simulink subsystem "Shrimple_6dof"  (R2023b)
settings: Solver=VariableStepAuto  StartTime=0.0  StopTime=10.0  RelTol=1e-3
undefined symbols (not defined in the file): Apogee_stop, BG0, Burnout_stop, COM_table, day_seconds, F, HG0, I, include_turbulence, latlong0, launch_elevation, Light, m_table, MIL, MOI_table, time0, turbulence_noise_seeds, uvw0_B, v0_NED, w0_BN, wind_model_type, x0_NED
libraries: sharedtransform x4, simulink_extras x2, aerolibwind2 x1
settings Model: Creator=thatf  LastModifiedBy=thatf

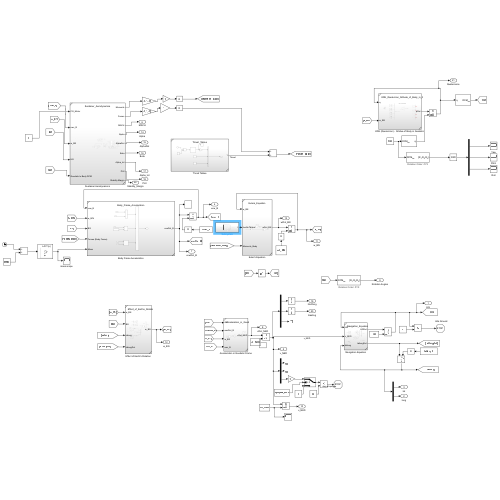
[thumbnail: Simulink's stored preview of the top-level diagram]
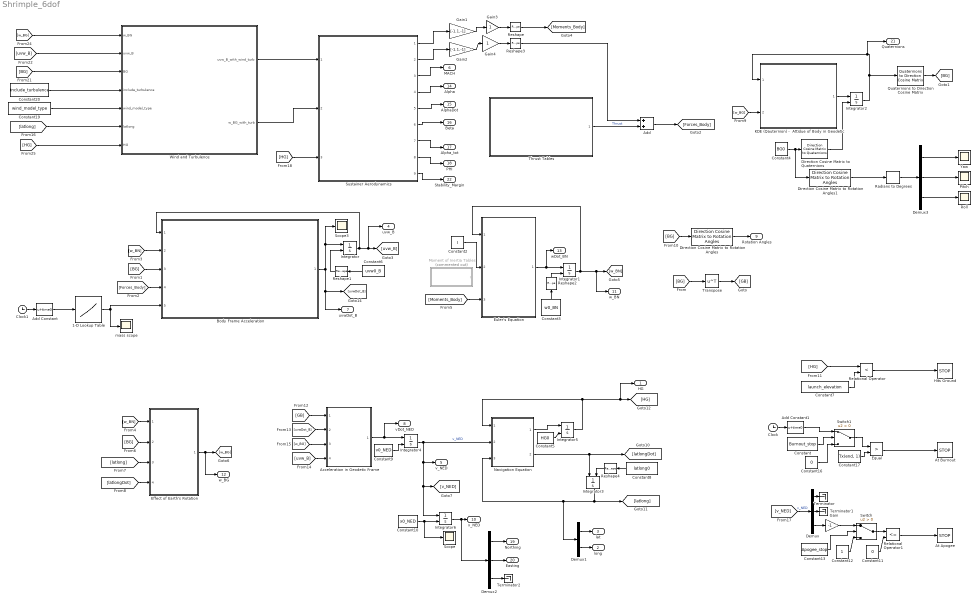
== system Shrimple_6dof ==
  1-D Lookup Table : Lookup_n-D  NumberOfTableDimensions=1  BreakpointsForDimension1=m_table(:,1)  Table=m_table(:,2)  InternalRulePriority=Speed  RndMeth=Simplest
  Acceleration in Geodetic Frame : Subsystem  ReferencedSubsystem=Acceleration_in_Geodetic_Frame
  Add : Sum
  Add Constant : Bias  Bias=time0  SaturateOnIntegerOverflow=off
  Add Constant1 : Bias  Bias=time0  SaturateOnIntegerOverflow=off
  At Apogee : Stop
  At Burnout : Stop
  Body Frame Acceleration : Subsystem  ReferencedSubsystem=Body_Frame_Acceleration
  Clock : Clock
  Clock1 : Clock
  Constant : Constant  Value=Burnout_stop
  Constant10 : Constant  Value=x0_NED
  Constant11 : Constant  Value=0
  Constant12 : Constant
  Constant13 : Constant  Value=Apogee_stop
  Constant16 : Constant  Value=0
  Constant17 : Constant  Value=Tx(end, 1)
  Constant19 : Constant  Value=wind_model_type
  Constant2 : Constant  Value=I
  Constant20 : Constant  Value=include_turbulence
  Constant3 : Constant  Value=w0_BN
  Constant4 : Constant  Value=BG0
  Constant5 : Constant  Value=HG0
  Constant6 : Constant  Value=uvw0_B
  Constant7 : Constant  Value=launch_elevation
  Constant8 : Constant  Value=latlong0
  Constant9 : Constant  Value=v0_NED
  Demux : Demux  Outputs=3
  Demux1 : Demux  Outputs=2
  Demux2 : Demux  Outputs=3
  Demux3 : Demux  Outputs=3
  Direction Cosine Matrix to Rotation Angles : sharedtransform/Direction Cosine Matrix to Rotation Angles  rotationOrder=ZYX  aMode=aMode  action=None  tolerance=eps(2)
  Direction Cosine Matrix to Rotation Angles1 : sharedtransform/Direction Cosine Matrix to Rotation Angles  rotationOrder=ZYX  aMode=aMode  action=None  tolerance=eps(2)
  Direction Cosine Matrix to Quaternions : sharedtransform/Direction Cosine Matrix  to Quaternions  aMode=0  action=None  tolerance=eps(2)
  Effect of Earth's Rotation : Subsystem  ReferencedSubsystem=Effect_of_Earths_Rotation
  Equal : RelationalOperator  Operator=>  OutDataTypeStr=boolean  RndMeth=Simplest  InputSameDT=off
  Euler's Equation : Subsystem  ReferencedSubsystem=Eulers_Equation
  Gain : Gain  Gain=-1
  Gain1 : Gain  Gain=[-1,1,-1]
  Gain2 : Gain  Gain=[-1,1,-1]
  Gain3 : Gain
  Gain4 : Gain
  Hits Ground : Stop
  Integrator{,1..6} (7 alike) : Integrator  InitialConditionSource=external
  "KDE (Qauternion) -  Attidue of Body in Geodetic " : Subsystem  ReferencedSubsystem=KDE_Qauternion_Attitude_of_Body_in_Geodetic
  Moment of Inertia Tables : Subsystem  Commented=on
  Navigation Equation : Subsystem  ReferencedSubsystem=Navigation_Equation
  Pitch : Scope
  Quaternions to Direction Cosine Matrix : sharedtransform/Quaternions to  Direction Cosine Matrix  aMode=aMode
  Radians to Degrees : simulink_extras/Transformations/Radians to Degrees
  Relational Operator : RelationalOperator  Operator=<  OutDataTypeStr=boolean  RndMeth=Simplest  InputSameDT=off
  Relational Operator1 : RelationalOperator  Operator=<=  OutDataTypeStr=boolean  RndMeth=Simplest  InputSameDT=off
  Reshape{,1..3} (4 alike) : Reshape  OutputDimensionality=Customize  OutputDimensions=[3,1]
  Reshape4 : Reshape  OutputDimensionality=Customize  OutputDimensions=[2,1]
  Roll : Scope
  Scope : Scope
  Scope3 : Scope
  Sustainer Aerodynamics : Subsystem  ReferencedSubsystem=Sustainer_Aerodynamics
  Switch : Switch  Criteria=u2 > Threshold  SaturateOnIntegerOverflow=off  InputSameDT=off
  Switch1 : Switch  Criteria=u2 > Threshold  SaturateOnIntegerOverflow=off  InputSameDT=off
  Terminator : Terminator
  Terminator1 : Terminator
  Terminator2 : Terminator
  Thrust Tables : Subsystem  ReferencedSubsystem=Thrust_Tables
  Transpose : Math  Operator=transpose
  Wind and Turbulence : Subsystem
  Yaw : Scope
  mass scope : Scope
  HG : Outport
  long : Outport  Port=2
  lat : Outport  Port=3
  uvw_B : Outport  Port=4
  v_NED : Outport  Port=5
  MACH : Outport  Port=6
  uvwDot_B : Outport  Port=7
  vDot_NED : Outport  Port=8
  Rotation Angles : Outport  Port=9
  x_NED : Outport  Port=10
  w_BN : Outport  Port=11
  w_BG : Outport  Port=12
  wDot_BN : Outport  Port=13
  Alpha : Outport  Port=14
  AlphaDot : Outport  Port=15
  Beta : Outport  Port=16
  Alpha_tot : Outport  Port=17
  PHI : Outport  Port=18
  Northing : Outport  Port=19
  Easting : Outport  Port=20
  Quaternions : Outport  Port=21
  Stability_Margin : Outport  Port=22
  wires:
  Euler's Equation/1 -> Integrator1/1, wDot_BN/1
  Direction Cosine Matrix to Rotation Angles/1 -> Rotation Angles/1
  [BG] -> Direction Cosine Matrix to Rotation Angles/1
  Direction Cosine Matrix to Quaternions/1 -> Integrator2/2
  Constant5/1 -> Integrator5/2
  [BG] -> Transpose/1
  [BG] -> Body Frame Acceleration/3
  [w_BG] -> Acceleration in Geodetic Frame/3
  Reshape/1 -> [Moments_Body]
  Constant6/1 -> Reshape1/1
  Navigation Equation/2 -> Integrator3/1, [latlongDot]
  Integrator2/1 -> Quaternions to Direction Cosine Matrix/1, "KDE (Qauternion) -  Attidue of Body in Geodetic "/1, Quaternions/1
  Constant3/1 -> Reshape2/1
  [BG] -> Effect of Earth's Rotation/2
  [uvw_B] -> Acceleration in Geodetic Frame/4
  [w_BG] -> "KDE (Qauternion) -  Attidue of Body in Geodetic "/2
  Reshape2/1 -> Integrator1/2
  Reshape1/1 -> Integrator/2
  Integrator3/1 -> Navigation Equation/3, Demux1/1, [latlong]
  Acceleration in Geodetic Frame/1 -> Integrator4/1, vDot_NED/1
  Body Frame Acceleration/1 -> Integrator/1, Scope3/1, [uvwDot_B], uvwDot_B/1
  Gain1/1 -> Gain3/1
  Navigation Equation/1 -> Integrator5/1
  Constant4/1 -> Direction Cosine Matrix to Quaternions/1, Direction Cosine Matrix to Rotation Angles1/1
  Integrator5/1 -> Navigation Equation/1, [HG], HG/1
  Gain2/1 -> Gain4/1
  "KDE (Qauternion) -  Attidue of Body in Geodetic "/1 -> Integrator2/1
  [Moments_Body] -> Euler's Equation/3
  [w_BN] -> Effect of Earth's Rotation/1
  Integrator4/1 -> v_NED/1, [v_NED], Integrator6/1, Navigation Equation/2  "v_NED"
  [w_BN] -> Body Frame Acceleration/2
  Integrator/1 -> Body Frame Acceleration/1, [uvw_B], uvw_B/1
  Quaternions to Direction Cosine Matrix/1 -> [BG]
  [uvwDot_B] -> Acceleration in Geodetic Frame/2
  Effect of Earth's Rotation/1 -> [w_BG], w_BG/1
  [GB] -> Acceleration in Geodetic Frame/1
  Transpose/1 -> [GB]
  Relational Operator/1 -> Hits Ground/1
  [Forces_Body] -> Body Frame Acceleration/4
  [latlongDot] -> Effect of Earth's Rotation/4
  Constant7/1 -> Relational Operator/2
  [latlong] -> Effect of Earth's Rotation/3
  Constant9/1 -> Integrator4/2
  Reshape4/1 -> Integrator3/2
  Integrator1/1 -> Euler's Equation/1, [w_BN], w_BN/1
  Constant8/1 -> Reshape4/1
  Demux1/2 -> long/1
  Demux1/1 -> lat/1
  Constant10/1 -> Integrator6/2, Scope/1
  Integrator6/1 -> x_NED/1, Demux2/1
  Reshape3/1 -> Add/1
  Thrust Tables/1 -> Add/2  "Thrust"
  Add/1 -> [Forces_Body]
  1-D Lookup Table/1 -> Body Frame Acceleration/5, mass scope/1
  Gain3/1 -> Reshape/1
  Gain4/1 -> Reshape3/1
  Demux2/3 -> Terminator2/1
  Direction Cosine Matrix to Rotation Angles1/1 -> Radians to Degrees/1
  Demux3/3 -> Roll/1
  Demux3/2 -> Pitch/1
  Radians to Degrees/1 -> Demux3/1
  Demux3/1 -> Yaw/1
  Sustainer Aerodynamics/8 -> PHI/1
  Sustainer Aerodynamics/7 -> Alpha_tot/1
  Sustainer Aerodynamics/6 -> Beta/1
  Sustainer Aerodynamics/5 -> AlphaDot/1
  Sustainer Aerodynamics/4 -> Alpha/1
  Sustainer Aerodynamics/3 -> MACH/1
  Sustainer Aerodynamics/2 -> Gain2/1
  Sustainer Aerodynamics/1 -> Gain1/1
  [HG] -> Sustainer Aerodynamics/3
  Sustainer Aerodynamics/9 -> Stability_Margin/1
  Equal/1 -> At Burnout/1
  Constant/1 -> Switch1/2
  Constant16/1 -> Switch1/3
  Constant17/1 -> Equal/2
  Switch1/1 -> Equal/1
  Add Constant1/1 -> Switch1/1
  Constant2/1 -> Euler's Equation/2
  Demux2/1 -> Northing/1
  Demux2/2 -> Easting/1
  [w_BG] -> Wind and Turbulence/1(w_BG)
  [uvw_B] -> Wind and Turbulence/2(uvw_B)
  [BG] -> Wind and Turbulence/3(BG)
  Constant20/1 -> Wind and Turbulence/4(include_turbulence)
  Constant19/1 -> Wind and Turbulence/5(wind_model_type)
  [latlong] -> Wind and Turbulence/6(latlong)
  [HG] -> Wind and Turbulence/7(HG)
  Wind and Turbulence/1(uvw_B_with_wind_turb) -> Sustainer Aerodynamics/1
  Wind and Turbulence/2(w_BG_with_turb) -> Sustainer Aerodynamics/2
  Clock1/1 -> Add Constant/1
  Add Constant/1 -> 1-D Lookup Table/1
  Clock/1 -> Add Constant1/1
  [HG] -> Relational Operator/1
  [v_NED] -> Demux/1  "v_NED"
  Demux/1 -> Terminator/1
  Constant13/1 -> Switch/2
  Gain/1 -> Switch/1
  Demux/3 -> Gain/1
  Constant12/1 -> Switch/3
  Switch/1 -> Relational Operator1/1
  Demux/2 -> Terminator1/1
  Constant11/1 -> Relational Operator1/2
  Relational Operator1/1 -> At Apogee/1

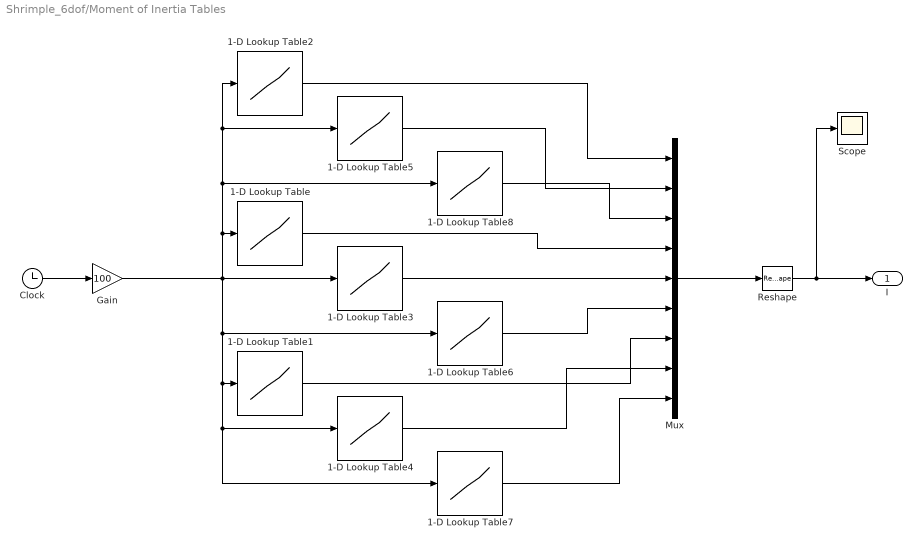
== system Shrimple_6dof/Moment of Inertia Tables ==
  1-D Lookup Table : Lookup_n-D  NumberOfTableDimensions=1  BreakpointsForDimension1=COM_table(:,1)  Table=MOI_table(:,2,1)  InternalRulePriority=Speed  RndMeth=Simplest
  1-D Lookup Table1 : Lookup_n-D  NumberOfTableDimensions=1  BreakpointsForDimension1=COM_table(:,1)  Table=MOI_table(:,3,1)  InternalRulePriority=Speed  RndMeth=Simplest
  1-D Lookup Table2 : Lookup_n-D  NumberOfTableDimensions=1  BreakpointsForDimension1=COM_table(:,1)  Table=MOI_table(:,1,1)  InternalRulePriority=Speed  RndMeth=Simplest
  1-D Lookup Table3 : Lookup_n-D  NumberOfTableDimensions=1  BreakpointsForDimension1=COM_table(:,1)  Table=MOI_table(:,2,2)  InternalRulePriority=Speed  RndMeth=Simplest
  1-D Lookup Table4 : Lookup_n-D  NumberOfTableDimensions=1  BreakpointsForDimension1=COM_table(:,1)  Table=MOI_table(:,3,2)  InternalRulePriority=Speed  RndMeth=Simplest
  1-D Lookup Table5 : Lookup_n-D  NumberOfTableDimensions=1  BreakpointsForDimension1=COM_table(:,1)  Table=MOI_table(:,1,2)  InternalRulePriority=Speed  RndMeth=Simplest
  1-D Lookup Table6 : Lookup_n-D  NumberOfTableDimensions=1  BreakpointsForDimension1=COM_table(:,1)  Table=MOI_table(:,2,3)  InternalRulePriority=Speed  RndMeth=Simplest
  1-D Lookup Table7 : Lookup_n-D  NumberOfTableDimensions=1  BreakpointsForDimension1=COM_table(:,1)  Table=MOI_table(:,3,3)  InternalRulePriority=Speed  RndMeth=Simplest
  1-D Lookup Table8 : Lookup_n-D  NumberOfTableDimensions=1  BreakpointsForDimension1=COM_table(:,1)  Table=MOI_table(:,1,3)  InternalRulePriority=Speed  RndMeth=Simplest
  Clock : Clock
  Gain : Gain  Gain=100
  Mux : Mux  Inputs=9
  Reshape : Reshape  OutputDimensionality=Customize  OutputDimensions=[3,3]
  Scope : Scope
  I : Outport
  wires:
  Gain/1 -> 1-D Lookup Table6/1, 1-D Lookup Table1/1, 1-D Lookup Table4/1, 1-D Lookup Table7/1, 1-D Lookup Table3/1, 1-D Lookup Table/1, 1-D Lookup Table8/1, 1-D Lookup Table5/1, 1-D Lookup Table2/1
  Reshape/1 -> I/1, Scope/1
  Mux/1 -> Reshape/1
  1-D Lookup Table7/1 -> Mux/9
  1-D Lookup Table4/1 -> Mux/8
  1-D Lookup Table1/1 -> Mux/7
  1-D Lookup Table6/1 -> Mux/6
  1-D Lookup Table3/1 -> Mux/5
  1-D Lookup Table/1 -> Mux/4
  1-D Lookup Table8/1 -> Mux/3
  1-D Lookup Table5/1 -> Mux/2
  1-D Lookup Table2/1 -> Mux/1
  Clock/1 -> Gain/1

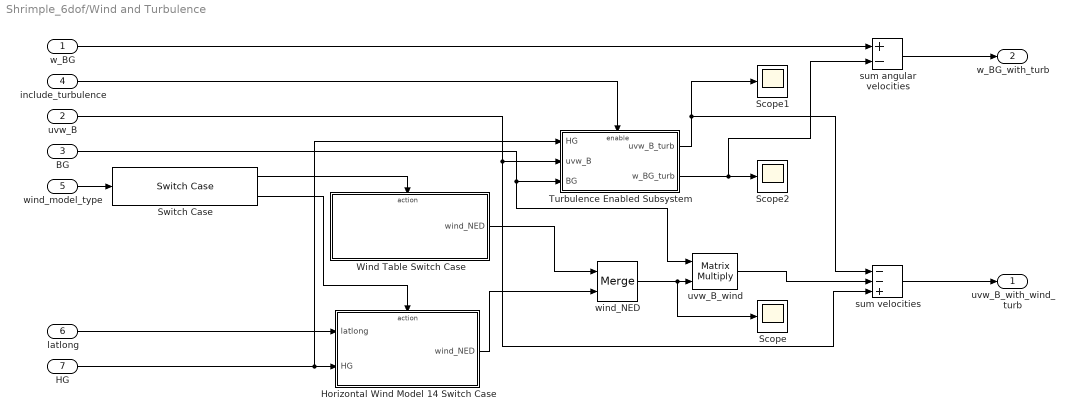
== system Shrimple_6dof/Wind and Turbulence ==
  w_BG : Inport
  uvw_B : Inport  Port=2
  BG : Inport  Port=3
  include_turbulence : Inport  Port=4
  wind_model_type : Inport  Port=5
  latlong : Inport  Port=6
  HG : Inport  Port=7
  Horizontal Wind Model 14 Switch Case : Subsystem  TreatAsAtomicUnit=on
  Scope : Scope
  Scope1 : Scope
  Scope2 : Scope
  Switch Case : SwitchCase  CaseConditions={WindModelType.WindTable, WindModelType.HorizontalWindModel14}  ShowDefaultCase=off
  Turbulence Enabled Subsystem : Subsystem  TreatAsAtomicUnit=on
  Wind Table Switch Case : Subsystem  TreatAsAtomicUnit=on
  sum angular velocities : Sum  Inputs=+-
  sum velocities : Sum  Inputs=--+
  uvw_B_wind : Product  Multiplication=Matrix(*)
  wind_NED : Merge
  uvw_B_with_wind_turb : Outport
  w_BG_with_turb : Outport  Port=2
  wires:
  Turbulence Enabled Subsystem/1(uvw_B_turb) -> sum velocities/1, Scope1/1
  Turbulence Enabled Subsystem/2(w_BG_turb) -> Scope2/1, sum angular velocities/2
  include_turbulence/1 -> Turbulence Enabled Subsystem/Enable
  sum velocities/1 -> uvw_B_with_wind_turb/1
  wind_model_type/1 -> Switch Case/1
  Switch Case/1 -> Wind Table Switch Case/Action
  uvw_B_wind/1 -> sum velocities/2
  Wind Table Switch Case/1(wind_NED) -> wind_NED/1
  w_BG/1 -> sum angular velocities/1
  Horizontal Wind Model 14 Switch Case/1(wind_NED) -> wind_NED/2
  latlong/1 -> Horizontal Wind Model 14 Switch Case/1(latlong)
  wind_NED/1 -> uvw_B_wind/2, Scope/1
  uvw_B/1 -> Turbulence Enabled Subsystem/2(uvw_B), sum velocities/3
  HG/1 -> Horizontal Wind Model 14 Switch Case/2(HG), Turbulence Enabled Subsystem/1(HG)
  Switch Case/2 -> Horizontal Wind Model 14 Switch Case/Action
  sum angular velocities/1 -> w_BG_with_turb/1
  BG/1 -> Turbulence Enabled Subsystem/3(BG), uvw_B_wind/1

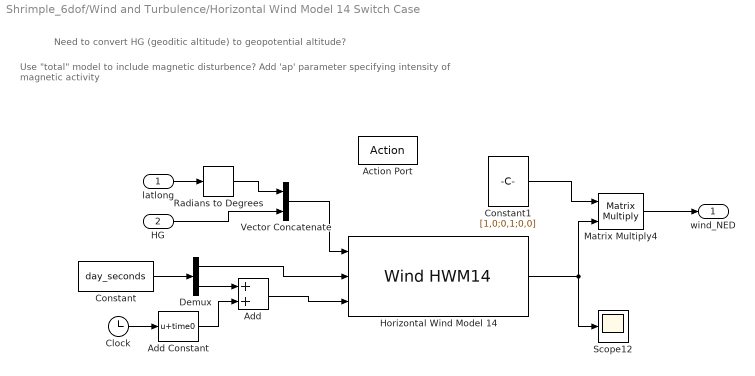
== system Shrimple_6dof/Wind and Turbulence/Horizontal Wind Model 14 Switch Case ==
  note: Need to convert HG (geoditic altitude) to geopotential altitude?
  note: Use "total" model to include magnetic disturbence? Add 'ap' parameter specifying intensity of magnetic activity
  latlong : Inport
  HG : Inport  Port=2
  Action Port : ActionPort
  Add : Sum
  Add Constant : Bias  Bias=time0  SaturateOnIntegerOverflow=off
  Clock : Clock
  Constant : Constant  Value=day_seconds
  Constant1 : Constant  Value=[1,0;0,1;0,0]
  Demux : Demux  Outputs=2
  Horizontal Wind Model 14 : WindHWM14
  Matrix Multiply4 : Product  Multiplication=Matrix(*)
  Radians to Degrees : simulink_extras/Transformations/Radians to Degrees
  Scope12 : Scope
  Vector Concatenate : Concatenate
  wind_NED : Outport
  wires:
  Add Constant/1 -> Add/2
  Clock/1 -> Add Constant/1
  Demux/2 -> Add/1
  Demux/1 -> Horizontal Wind Model 14/2
  Constant/1 -> Demux/1
  Matrix Multiply4/1 -> wind_NED/1
  Constant1/1 -> Matrix Multiply4/1
  Horizontal Wind Model 14/1 -> Scope12/1, Matrix Multiply4/2
  Vector Concatenate/1 -> Horizontal Wind Model 14/1
  HG/1 -> Vector Concatenate/2
  Radians to Degrees/1 -> Vector Concatenate/1
  latlong/1 -> Radians to Degrees/1
  Add/1 -> Horizontal Wind Model 14/3

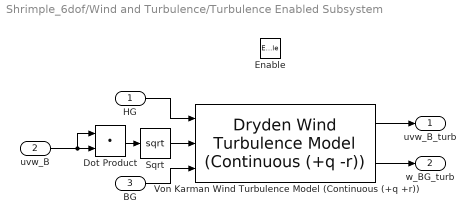
== system Shrimple_6dof/Wind and Turbulence/Turbulence Enabled Subsystem ==
  HG : Inport
  uvw_B : Inport  Port=2
  BG : Inport  Port=3
  Enable : EnablePort
  Dot Product : DotProduct  OutDataTypeStr=Inherit: Inherit via internal rule
  Sqrt : Sqrt
  Von Karman Wind Turbulence Model (Continuous (+q +r)) : aerolibwind2/Dryden Wind Turbulence Model  (Continuous (+q -r))  units=Metric (MKS)  spec=MIL-F-8785C  model=Continuous Von Karman (+q +r)  W20=wind_speed6m  Wdeg=wind_direction6m  TurbProb=10^-2 - Light  L_high=762  Wingspan=finspan  ts=0.1  Seed=turbulence_noise_seeds  T_on=on
      settings: LibrarySourceBlock=|
      | aerolibwind2/Von Karman Wind Turbulence Model
      | (Continuous (+q +r))
  uvw_B_turb : Outport
  w_BG_turb : Outport  Port=2
  wires:
  Von Karman Wind Turbulence Model (Continuous (+q +r))/2 -> w_BG_turb/1
  HG/1 -> Von Karman Wind Turbulence Model (Continuous (+q +r))/1
  Von Karman Wind Turbulence Model (Continuous (+q +r))/1 -> uvw_B_turb/1
  BG/1 -> Von Karman Wind Turbulence Model (Continuous (+q +r))/3
  Dot Product/1 -> Sqrt/1
  uvw_B/1 -> Dot Product/2, Dot Product/1
  Sqrt/1 -> Von Karman Wind Turbulence Model (Continuous (+q +r))/2

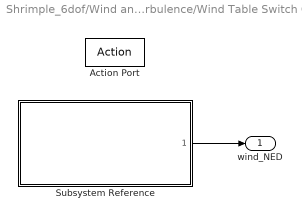
== system Shrimple_6dof/Wind and Turbulence/Wind Table Switch Case ==
  Action Port : ActionPort
  Subsystem Reference : Subsystem  ReferencedSubsystem=Wind_Table
  wind_NED : Outport
  wires:
  Subsystem Reference/1 -> wind_NED/1
